simulink model "networkanalyzer"  (R2012b)
settings: Solver=ode3  SolverMode=SingleTasking  StartTime=0.0  StopTime=50000  RelTol=1e-3
libraries: xbsIndex_r4 x1097, casper_library_flow_control x33, casper_library_misc x21, xps_library x10
(part 1 of 8)
settings Model: Creator=tmadden  LastModifiedBy=tmadden

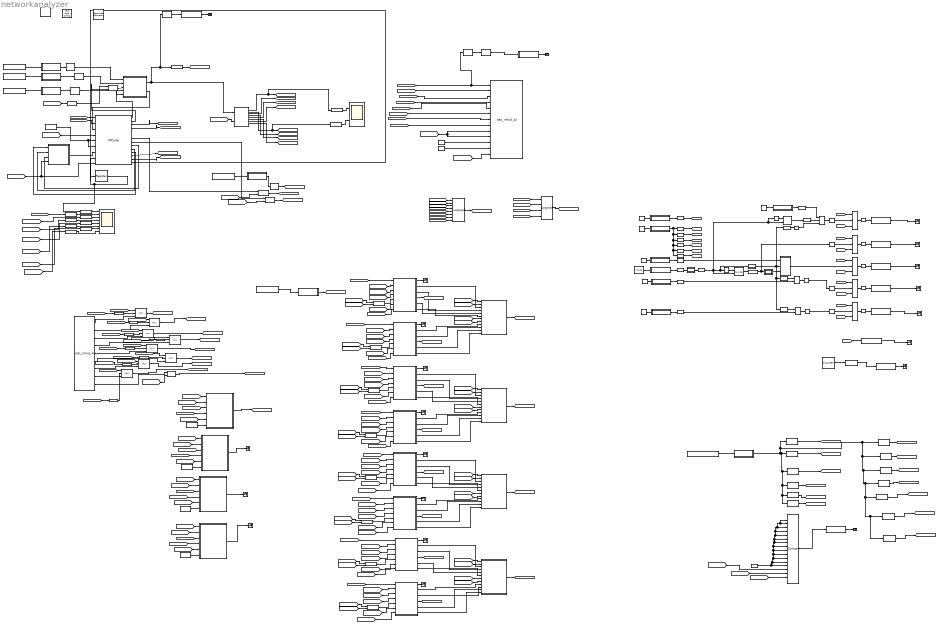
== system networkanalyzer ==
  note: The above is Ran's design for  ROACH IF baord
      | serial data stream. For programming IF board
      | clocks, gains, dividers.
  note: Signed 8 bit int
  note: Signed 8 bit, integer
  note: acc_cntrl has a clock
      | cycle latency in generating
      | new_acc signal.
      | Compensate by delaying
      | ata here.
  note: SWAT_LE
  note: LO_SLE
  note: SER_DI
  note: SER_CLK
  note: SW_STB
  note: Added by Tim Madden
  note: not in RANS design- below. Tim added the clk sle register so we can program the clocks
  note: bit 7
  note: CLK_SLE
  " System Generator" : xbsIndex_r4/ System Generator  Tag=genX  xilinxfamily=virtex5  part=xc5vsx95t  speed=-1  package=ff1136  synthesis_tool=XST  clock_wrapper=Clock Enables  directory=./networkanalyzer/sysgen  proj_type=Project Navigator  Synth_file=XST Defaults  Impl_file=ISE Defaults  testbench=off  simulink_period=1  sysclk_period=7.8125  dcm_input_clock_period=100  incr_netlist=off  trim_vbits=Everywhere in SubSystem  dbl_ovrd=According to Block Masks  core_generation=According to Block Masks  run_coregen=off  deprecated_control=off  eval_field=0  block_type=sysgen
  Concat : xbsIndex_r4/Concat  num_inputs=16  dbl_ovrd=off  block_type=concat
  Constant{,17..19} (4 alike) : xbsIndex_r4/Constant  const=0  gui_display_data_type=Boolean  arith_type=Boolean  n_bits=16  bin_pt=14  preci_type=Single  exp_width=8  frac_width=24  explicit_period=on  period=1  equ=P=C  opselect=C  inp2=PCIN>>17  opr=+  inp1=P  carry=CIN  dbl_ovrd=off  block_type=constant
  Constant1 : Constant  Value=(2^1) + (2^3) + (2^4) + (2^9)+(2^12)
  Constant10 : xbsIndex_r4/Constant  const=0  gui_display_data_type=Boolean  arith_type=Boolean  n_bits=4  bin_pt=0  preci_type=Single  exp_width=8  frac_width=24  explicit_period=on  period=1  equ=P=C  opselect=C  inp2=PCIN>>17  opr=+  inp1=P  carry=CIN  dbl_ovrd=off  block_type=constant
      settings: block_version=11.4
  Constant{11,13..15} (4 alike) : Constant
  Constant12 : Constant  Value=2^31 + 2^29 + 2^15+2^4 + 2^0
  Constant16 : Constant  Value=0
  Constant2 : Constant  Value=83886080
  Constant20 : Constant  Value=(2^26)*(64/512)
  Constant3 : Constant  Value=838860800
  Constant4 : Constant  Value=368640
  Constant5 : xbsIndex_r4/Constant  const=0  gui_display_data_type=Boolean  arith_type=Boolean  n_bits=16  bin_pt=14  preci_type=Single  exp_width=8  frac_width=24  explicit_period=off  period=1  equ=P=C  opselect=C  inp2=PCIN>>17  opr=+  inp1=P  carry=CIN  dbl_ovrd=off  block_type=constant
  Constant6 : xbsIndex_r4/Constant  const=0  gui_display_data_type=Fixed-point  arith_type=Boolean  n_bits=4  bin_pt=0  preci_type=Single  exp_width=8  frac_width=24  explicit_period=on  period=1  equ=P=C  opselect=C  inp2=PCIN>>17  opr=+  inp1=P  carry=CIN  dbl_ovrd=off  block_type=constant
      settings: block_version=11.4
  Constant8 : xbsIndex_r4/Constant  const=0  gui_display_data_type=Fixed-point  arith_type=Unsigned  n_bits=4  bin_pt=0  preci_type=Single  exp_width=8  frac_width=24  explicit_period=on  period=1  equ=P=C  opselect=C  inp2=PCIN>>17  opr=+  inp1=P  carry=CIN  dbl_ovrd=off  block_type=constant
      settings: block_version=11.4
  Constant9 : Constant  Value=512
  Convert : xbsIndex_r4/Convert  gui_display_data_type=Fixed-point  arith_type="Signed  (2's comp)"  n_bits=32  bin_pt=15  float_type=Single  exp_bits=8  fraction_bits=24  quantization=Truncate  overflow=Wrap  en=off  latency=0  dbl_ovrd=off  pipeline=off  block_type=convert
  Convert5 : xbsIndex_r4/Convert  gui_display_data_type=Fixed-point  arith_type=Unsigned  n_bits=33  bin_pt=0  float_type=Single  exp_bits=8  fraction_bits=24  quantization=Truncate  overflow=Wrap  en=off  latency=0  dbl_ovrd=off  pipeline=off  block_type=convert
      settings: block_version=11.4
  CosSinGen : Subsystem
  Counter : xbsIndex_r4/Counter  cnt_type=Free Running  cnt_to=Inf  operation=Up  start_count=0  cnt_by_val=1  arith_type=Unsigned  n_bits=24  bin_pt=0  load_pin=off  rst=off  en=off  explicit_period=on  period=1  dbl_ovrd=off  use_behavioral_HDL=off  implementation=Fabric  block_type=counter
  Counter2 : xbsIndex_r4/Counter  cnt_type=Free Running  cnt_to=2048  operation=Up  start_count=0  cnt_by_val=1  arith_type=Unsigned  n_bits=8  bin_pt=0  load_pin=off  rst=on  en=on  explicit_period=on  period=1  dbl_ovrd=off  use_behavioral_HDL=off  implementation=Fabric  use_rpm=off  block_type=counter
  Counter4 : xbsIndex_r4/Counter  cnt_type=Free Running  cnt_to=Inf  operation=Up  start_count=0  cnt_by_val=1  arith_type=Unsigned  n_bits=8  bin_pt=0  load_pin=off  rst=on  en=on  explicit_period=on  period=1  dbl_ovrd=off  use_behavioral_HDL=off  implementation=Fabric  block_type=counter
      settings: block_version=11.4
  DFTMem1 : Subsystem
  DFTMem2 : Subsystem
  DFTMem3 : Subsystem
  DFTMem4 : Subsystem
  DFTW : Subsystem
  DFTW1 : Subsystem
  DFTW2 : Subsystem
  DFTW3 : Subsystem
  DFTW4 : Subsystem
  DFTW5 : Subsystem
  DFTW6 : Subsystem
  DFTW7 : Subsystem
  Delay{1..2,9..12,29..32,34} (11 alike) : xbsIndex_r4/Delay  rst=off  infoeditControl=Selection of Reset will increase slice count due to use of real FFs and instead of SRLs  en=off  latency=1  dbl_ovrd=off  reg_retiming=off  block_type=delay
  Delay{23..24,27..28} (4 alike) : xbsIndex_r4/Delay  rst=off  infoeditControl=Selection of Reset will increase slice count due to use of real FFs and instead of SRLs  en=off  latency=64  dbl_ovrd=off  reg_retiming=off  block_type=delay
      settings: block_version=11.4
  FreqSweeper : Subsystem
  Gateway Out{1..5,7..8,12..15} (11 alike) : xbsIndex_r4/Gateway Out  inherit_from_input=off  hdl_port=off  timing_constraint=None  locs_specified=off  LOCs={}  UseAsDAC=off  DACChannel='1'  block_type=gatewayout
  Inverter{1..5} (5 alike) : xbsIndex_r4/Inverter  en=off  latency=0  dbl_ovrd=off  block_type=inv
      settings: block_version=11.4
  LO_SLE : Subsystem  Tag=xps:sw_reg  AncestorBlock=xps_library/software register  mask{numios=1, io_dir=From Processor, io_delay=0, sample_period=1, name1=reg, bitwidth1=32, arith_type1=Unsigned, bin_pt1=0}
      mask prompts: numios "Num I/Os"; io_dir "I/O direction"; io_delay "I/O delay"; sample_period "Sample period"; name1 "Name"; bitwidth1 "Bitwidth"; arith_type1 "Type"; bin_pt1 "Binary pt"
      mask init:
      | swreg_init(gcb);
      mask Callback numios: t = timer('StartDelay', 0.1); t.TimerFcn = {@swreg_cb, gcb}; start(t);
      mask TypeOptions io_dir: To Processor | From Processor
      mask Callback io_dir:
      | a = get_param(gcb, 'MaskEnables');
      | if strcmp(get_param(gcb, 'io_dir'), 'To Processor'),
      | a(4) = {'off'};
      | else
      | a(4) = {'on'};
      | end
      | set_param(gcb, 'MaskEnables', a);
      mask TypeOptions arith_type1: Unsigned | Signed  (2's comp) | Boolean
      mask Callback arith_type1:
      | a = get_param(gcb, 'MaskEnables');
      | if strcmp(get_param(gcb, 'arith_type1'), 'Boolean'),
      | set_param(gcb, 'bitwidth1', '1');
      | set_param(gcb, 'bin_pt1', '0');
      | a(6) = {'off'};
      | a(8) = {'off'};
      | else
      | a(6) = {'on'};
      | a(8) = {'on'};
      | end
      | set_param(gcb, 'MaskEnables', a);
  Logical{,1..2,17} (4 alike) : xbsIndex_r4/Logical  logical_function=OR  inputs=2  en=off  latency=0  precision=Full  arith_type=Unsigned  n_bits=16  bin_pt=0  align_bp=on  dbl_ovrd=off  block_type=logical
  Logical{3..8,10..13} (10 alike) : xbsIndex_r4/Logical  logical_function=AND  inputs=2  en=off  latency=0  precision=Full  arith_type=Unsigned  n_bits=16  bin_pt=0  align_bp=on  dbl_ovrd=off  block_type=logical
      Logical7 settings: block_version=11.4
      Logical8 settings: block_version=11.4
  Logical14 : xbsIndex_r4/Logical  logical_function=AND  inputs=8  en=off  latency=1  precision=Full  arith_type=Unsigned  n_bits=16  bin_pt=0  align_bp=on  dbl_ovrd=off  block_type=logical
  Logical15 : xbsIndex_r4/Logical  logical_function=AND  inputs=4  en=off  latency=1  precision=Full  arith_type=Unsigned  n_bits=16  bin_pt=0  align_bp=on  dbl_ovrd=off  block_type=logical
  Logical9 : xbsIndex_r4/Logical  logical_function=AND  inputs=3  en=off  latency=0  precision=Full  arith_type=Unsigned  n_bits=16  bin_pt=0  align_bp=on  dbl_ovrd=off  block_type=logical
      settings: block_version=11.4
  MainFSMScope1 : Scope  NumInputPorts=8
      settings: YMin=0~-5~-5~-5~-5~-5~-5~-5  YMax=300000~5~5~5~5~5~5~5  SaveName=ScopeData7  MaxDataPoints=10000
  MainFSMScope2 : Scope  NumInputPorts=2
      settings: YMin=0~-5  YMax=300000~5  SaveName=ScopeData2  MaxDataPoints=10000
  Mux{,1..12} (13 alike) : xbsIndex_r4/Mux  inputs=2  en=off  latency=1  precision=Full  arith_type=Unsigned  n_bits=16  bin_pt=14  quantization=Truncate  overflow=Wrap  dbl_ovrd=off  block_type=mux
      Mux2 settings: block_version=11.4
      Mux3 settings: block_version=11.4
      Mux4 settings: block_version=11.4
      Mux5 settings: block_version=11.4
      Mux6 settings: block_version=11.4
  Pulse Generator2 : DiscretePulseGenerator  Period=11000  PulseWidth=10000  PhaseDelay=100
  Resource Estimator : xbsIndex_r4/Resource Estimator  Tag=resEstTag  Slices=0  FFs=0  BRAMs=0  LUTs=0  IOBs=0  EBMs=0  TBUFs=0  xl_use_estimator_area=off  est_options=Estimate  xl_estimator_area=[392 0 0 632 0 0 0]  block_type=resource_estimator
      settings: AttributesFormatString=Resource\nEstimator
  SER_DI : Subsystem  Tag=xps:sw_reg  AncestorBlock=xps_library/software register  mask{numios=1, io_dir=From Processor, io_delay=0, sample_period=1, name1=reg, bitwidth1=32, arith_type1=Unsigned, bin_pt1=0}
      mask prompts: numios "Num I/Os"; io_dir "I/O direction"; io_delay "I/O delay"; sample_period "Sample period"; name1 "Name"; bitwidth1 "Bitwidth"; arith_type1 "Type"; bin_pt1 "Binary pt"
      mask init:
      | swreg_init(gcb);
      mask Callback numios: t = timer('StartDelay', 0.1); t.TimerFcn = {@swreg_cb, gcb}; start(t);
      mask TypeOptions io_dir: To Processor | From Processor
      mask Callback io_dir:
      | a = get_param(gcb, 'MaskEnables');
      | if strcmp(get_param(gcb, 'io_dir'), 'To Processor'),
      | a(4) = {'off'};
      | else
      | a(4) = {'on'};
      | end
      | set_param(gcb, 'MaskEnables', a);
      mask TypeOptions arith_type1: Unsigned | Signed  (2's comp) | Boolean
      mask Callback arith_type1:
      | a = get_param(gcb, 'MaskEnables');
      | if strcmp(get_param(gcb, 'arith_type1'), 'Boolean'),
      | set_param(gcb, 'bitwidth1', '1');
      | set_param(gcb, 'bin_pt1', '0');
      | a(6) = {'off'};
      | a(8) = {'off'};
      | else
      | a(6) = {'on'};
      | a(8) = {'on'};
      | end
      | set_param(gcb, 'MaskEnables', a);
  SWAT_LE : Subsystem  Tag=xps:sw_reg  AncestorBlock=xps_library/software register  mask{numios=1, io_dir=From Processor, io_delay=0, sample_period=1, name1=reg, bitwidth1=32, arith_type1=Unsigned, bin_pt1=0}
      mask prompts: numios "Num I/Os"; io_dir "I/O direction"; io_delay "I/O delay"; sample_period "Sample period"; name1 "Name"; bitwidth1 "Bitwidth"; arith_type1 "Type"; bin_pt1 "Binary pt"
      mask init:
      | swreg_init(gcb);
      mask Callback numios: t = timer('StartDelay', 0.1); t.TimerFcn = {@swreg_cb, gcb}; start(t);
      mask TypeOptions io_dir: To Processor | From Processor
      mask Callback io_dir:
      | a = get_param(gcb, 'MaskEnables');
      | if strcmp(get_param(gcb, 'io_dir'), 'To Processor'),
      | a(4) = {'off'};
      | else
      | a(4) = {'on'};
      | end
      | set_param(gcb, 'MaskEnables', a);
      mask TypeOptions arith_type1: Unsigned | Signed  (2's comp) | Boolean
      mask Callback arith_type1:
      | a = get_param(gcb, 'MaskEnables');
      | if strcmp(get_param(gcb, 'arith_type1'), 'Boolean'),
      | set_param(gcb, 'bitwidth1', '1');
      | set_param(gcb, 'bin_pt1', '0');
      | a(6) = {'off'};
      | a(8) = {'off'};
      | else
      | a(6) = {'on'};
      | a(8) = {'on'};
      | end
      | set_param(gcb, 'MaskEnables', a);
  SixFourDivLen32p26 : Subsystem  Tag=xps:sw_reg  AncestorBlock=xps_library/software register  mask{numios=1, io_dir=From Processor, io_delay=0, sample_period=1, name1=reg, bitwidth1=32, arith_type1=Unsigned, bin_pt1=0}
      mask prompts: numios "Num I/Os"; io_dir "I/O direction"; io_delay "I/O delay"; sample_period "Sample period"; name1 "Name"; bitwidth1 "Bitwidth"; arith_type1 "Type"; bin_pt1 "Binary pt"
      mask init:
      | swreg_init(gcb);
      mask Callback numios: t = timer('StartDelay', 0.1); t.TimerFcn = {@swreg_cb, gcb}; start(t);
      mask TypeOptions io_dir: To Processor | From Processor
      mask Callback io_dir:
      | a = get_param(gcb, 'MaskEnables');
      | if strcmp(get_param(gcb, 'io_dir'), 'To Processor'),
      | a(4) = {'off'};
      | else
      | a(4) = {'on'};
      | end
      | set_param(gcb, 'MaskEnables', a);
      mask TypeOptions arith_type1: Unsigned | Signed  (2's comp) | Boolean
      mask Callback arith_type1:
      | a = get_param(gcb, 'MaskEnables');
      | if strcmp(get_param(gcb, 'arith_type1'), 'Boolean'),
      | set_param(gcb, 'bitwidth1', '1');
      | set_param(gcb, 'bin_pt1', '0');
      | a(6) = {'off'};
      | a(8) = {'off'};
      | else
      | a(6) = {'on'};
      | a(8) = {'on'};
      | end
      | set_param(gcb, 'MaskEnables', a);
  Slice1 : xbsIndex_r4/Slice  nbits=1  boolean_output=on  mode=Lower Bit Location + Width  bit1=0  base1=MSB of Input  bit0=4  base0=LSB of Input  dbl_ovrd=off  block_type=slice
  Slice10 : xbsIndex_r4/Slice  nbits=1  boolean_output=on  mode=Upper Bit Location + Width  bit1=0  base1=MSB of Input  bit0=0  base0=LSB of Input  dbl_ovrd=off  block_type=slice
  Slice11 : xbsIndex_r4/Slice  nbits=1  boolean_output=on  mode=Lower Bit Location + Width  bit1=0  base1=MSB of Input  bit0=3  base0=LSB of Input  dbl_ovrd=off  block_type=slice
  Slice{14..15,20..21,26} (5 alike) : xbsIndex_r4/Slice  nbits=1  boolean_output=on  mode=Lower Bit Location + Width  bit1=0  base1=MSB of Input  bit0=0  base0=LSB of Input  dbl_ovrd=off  block_type=slice
  Slice2 : xbsIndex_r4/Slice  nbits=1  boolean_output=off  mode=Lower Bit Location + Width  bit1=0  base1=MSB of Input  bit0=0  base0=LSB of Input  dbl_ovrd=off  block_type=slice
  Slice22 : xbsIndex_r4/Slice  nbits=1  boolean_output=on  mode=Lower Bit Location + Width  bit1=0  base1=MSB of Input  bit0=1  base0=LSB of Input  dbl_ovrd=off  block_type=slice
  Slice25 : xbsIndex_r4/Slice  nbits=1  boolean_output=off  mode=Lower Bit Location + Width  bit1=0  base1=MSB of Input  bit0=2  base0=LSB of Input  dbl_ovrd=off  block_type=slice
  Slice3 : xbsIndex_r4/Slice  nbits=7  boolean_output=on  mode=Lower Bit Location + Width  bit1=0  base1=MSB of Input  bit0=0  base0=MSB of Input  dbl_ovrd=off  block_type=slice
      settings: block_version=10.1.3
  Slice4 : xbsIndex_r4/Slice  nbits=1  boolean_output=on  mode=Lower Bit Location + Width  bit1=0  base1=MSB of Input  bit0=5  base0=LSB of Input  dbl_ovrd=off  block_type=slice
  Stack4_ : Subsystem
  Terminator{,1..20} (21 alike) : Terminator
  XSG core config : xps_library/XSG core config  Tag=xps:xsg  hw_sys=ROACH:sx95t  clk_src=adc1_clk  ROACH_clk_src=adc1_clk  ROACH2_clk_src=adc0_clk  clk_rate=128  sample_period=1  synthesis_tool=XST
  adcWaveMem : Subsystem
  adcWaveMem1 : Subsystem
  adcWaveMem2 : Subsystem
  adcWaveMem3 : Subsystem
  adc_mkid_4x : xps_library/ADCs/adc_mkid_4x  Tag=xps:adc_mkid_4x  adc_brd=1  adc_clk_rate=512
  bit0 : xbsIndex_r4/Slice  nbits=1  boolean_output=on  mode=Lower Bit Location + Width  bit1=0  base1=MSB of Input  bit0=0  base0=LSB of Input  dbl_ovrd=off  block_type=slice
  bit1 : xbsIndex_r4/Slice  nbits=1  boolean_output=on  mode=Lower Bit Location + Width  bit1=0  base1=MSB of Input  bit0=1  base0=LSB of Input  dbl_ovrd=off  block_type=slice
  bit12 : xbsIndex_r4/Slice  nbits=1  boolean_output=on  mode=Lower Bit Location + Width  bit1=0  base1=MSB of Input  bit0=12  base0=LSB of Input  dbl_ovrd=off  block_type=slice
  bit13 : xbsIndex_r4/Slice  nbits=1  boolean_output=on  mode=Lower Bit Location + Width  bit1=0  base1=MSB of Input  bit0=13  base0=LSB of Input  dbl_ovrd=off  block_type=slice
  bit15 : xbsIndex_r4/Slice  nbits=1  boolean_output=on  mode=Lower Bit Location + Width  bit1=0  base1=MSB of Input  bit0=15  base0=LSB of Input  dbl_ovrd=off  block_type=slice
  bit2 : xbsIndex_r4/Slice  nbits=1  boolean_output=on  mode=Lower Bit Location + Width  bit1=0  base1=MSB of Input  bit0=2  base0=LSB of Input  dbl_ovrd=off  block_type=slice
  bit3 : xbsIndex_r4/Slice  nbits=1  boolean_output=on  mode=Lower Bit Location + Width  bit1=0  base1=MSB of Input  bit0=3  base0=LSB of Input  dbl_ovrd=off  block_type=slice
  bit4 : xbsIndex_r4/Slice  nbits=1  boolean_output=on  mode=Lower Bit Location + Width  bit1=0  base1=MSB of Input  bit0=4  base0=LSB of Input  dbl_ovrd=off  block_type=slice
  bit5 : xbsIndex_r4/Slice  nbits=1  boolean_output=on  mode=Lower Bit Location + Width  bit1=0  base1=MSB of Input  bit0=5  base0=LSB of Input  dbl_ovrd=off  block_type=slice
  bit6 : xbsIndex_r4/Slice  nbits=1  boolean_output=on  mode=Lower Bit Location + Width  bit1=0  base1=MSB of Input  bit0=6  base0=LSB of Input  dbl_ovrd=off  block_type=slice
  bit7 : xbsIndex_r4/Slice  nbits=1  boolean_output=on  mode=Lower Bit Location + Width  bit1=0  base1=MSB of Input  bit0=7  base0=LSB of Input  dbl_ovrd=off  block_type=slice
  bit8 : xbsIndex_r4/Slice  nbits=1  boolean_output=on  mode=Lower Bit Location + Width  bit1=0  base1=MSB of Input  bit0=8  base0=LSB of Input  dbl_ovrd=off  block_type=slice
  bit9__ : xbsIndex_r4/Slice  nbits=1  boolean_output=off  mode=Lower Bit Location + Width  bit1=0  base1=MSB of Input  bit0=9  base0=LSB of Input  dbl_ovrd=off  block_type=slice
  cntbit10 : xbsIndex_r4/Slice  nbits=1  boolean_output=off  mode=Lower Bit Location + Width  bit1=0  base1=LSB of Input  bit0=10  base0=LSB of Input  dbl_ovrd=off  block_type=slice
  controlReg : Subsystem  Tag=xps:sw_reg  AncestorBlock=xps_library/software register  mask{numios=1, io_dir=From Processor, io_delay=0, sample_period=1, name1=reg, bitwidth1=32, arith_type1=Unsigned, bin_pt1=0}
      mask prompts: numios "Num I/Os"; io_dir "I/O direction"; io_delay "I/O delay"; sample_period "Sample period"; name1 "Name"; bitwidth1 "Bitwidth"; arith_type1 "Type"; bin_pt1 "Binary pt"
      mask init:
      | swreg_init(gcb);
      mask Callback numios: t = timer('StartDelay', 0.1); t.TimerFcn = {@swreg_cb, gcb}; start(t);
      mask TypeOptions io_dir: To Processor | From Processor
      mask Callback io_dir:
      | a = get_param(gcb, 'MaskEnables');
      | if strcmp(get_param(gcb, 'io_dir'), 'To Processor'),
      | a(4) = {'off'};
      | else
      | a(4) = {'on'};
      | end
      | set_param(gcb, 'MaskEnables', a);
      mask TypeOptions arith_type1: Unsigned | Signed  (2's comp) | Boolean
      mask Callback arith_type1:
      | a = get_param(gcb, 'MaskEnables');
      | if strcmp(get_param(gcb, 'arith_type1'), 'Boolean'),
      | set_param(gcb, 'bitwidth1', '1');
      | set_param(gcb, 'bin_pt1', '0');
      | a(6) = {'off'};
      | a(8) = {'off'};
      | else
      | a(6) = {'on'};
      | a(8) = {'on'};
      | end
      | set_param(gcb, 'MaskEnables', a);
  currentFreq : Subsystem  Tag=xps:sw_reg  AncestorBlock=xps_library/software register  mask{numios=1, io_dir=To Processor, io_delay=0, sample_period=1, name1=reg, bitwidth1=32, arith_type1=Unsigned, bin_pt1=0}
      mask prompts: numios "Num I/Os"; io_dir "I/O direction"; io_delay "I/O delay"; sample_period "Sample period"; name1 "Name"; bitwidth1 "Bitwidth"; arith_type1 "Type"; bin_pt1 "Binary pt"
      mask init:
      | swreg_init(gcb);
      mask Callback numios: t = timer('StartDelay', 0.1); t.TimerFcn = {@swreg_cb, gcb}; start(t);
      mask TypeOptions io_dir: To Processor | From Processor
      mask Callback io_dir:
      | a = get_param(gcb, 'MaskEnables');
      | if strcmp(get_param(gcb, 'io_dir'), 'To Processor'),
      | a(4) = {'off'};
      | else
      | a(4) = {'on'};
      | end
      | set_param(gcb, 'MaskEnables', a);
      mask TypeOptions arith_type1: Unsigned | Signed  (2's comp) | Boolean
      mask Callback arith_type1:
      | a = get_param(gcb, 'MaskEnables');
      | if strcmp(get_param(gcb, 'arith_type1'), 'Boolean'),
      | set_param(gcb, 'bitwidth1', '1');
      | set_param(gcb, 'bin_pt1', '0');
      | a(6) = {'off'};
      | a(8) = {'off'};
      | else
      | a(6) = {'on'};
      | a(8) = {'on'};
      | end
      | set_param(gcb, 'MaskEnables', a);
  currentState : xbsIndex_r4/Register  init=0  rst=off  en=off  dbl_ovrd=off  block_type=register
  dac_mkid_4x : xps_library/DACs/dac_mkid_4x  Tag=xps:dac_mkid_4x  dac_brd=0  dac_clk_rate=512  sample_period=1
  dftLen : Subsystem  Tag=xps:sw_reg  AncestorBlock=xps_library/software register  mask{numios=1, io_dir=From Processor, io_delay=0, sample_period=1, name1=reg, bitwidth1=32, arith_type1=Unsigned, bin_pt1=0}
      mask prompts: numios "Num I/Os"; io_dir "I/O direction"; io_delay "I/O delay"; sample_period "Sample period"; name1 "Name"; bitwidth1 "Bitwidth"; arith_type1 "Type"; bin_pt1 "Binary pt"
      mask init:
      | swreg_init(gcb);
      mask Callback numios: t = timer('StartDelay', 0.1); t.TimerFcn = {@swreg_cb, gcb}; start(t);
      mask TypeOptions io_dir: To Processor | From Processor
      mask Callback io_dir:
      | a = get_param(gcb, 'MaskEnables');
      | if strcmp(get_param(gcb, 'io_dir'), 'To Processor'),
      | a(4) = {'off'};
      | else
      | a(4) = {'on'};
      | end
      | set_param(gcb, 'MaskEnables', a);
      mask TypeOptions arith_type1: Unsigned | Signed  (2's comp) | Boolean
      mask Callback arith_type1:
      | a = get_param(gcb, 'MaskEnables');
      | if strcmp(get_param(gcb, 'arith_type1'), 'Boolean'),
      | set_param(gcb, 'bitwidth1', '1');
      | set_param(gcb, 'bin_pt1', '0');
      | a(6) = {'off'};
      | a(8) = {'off'};
      | else
      | a(6) = {'on'};
      | a(8) = {'on'};
      | end
      | set_param(gcb, 'MaskEnables', a);
  edge_detect : casper_library_misc/edge_detect  edge=Rising  polarity=Active High  x_in=[0 0.08 0.08 0.16 0.16 0.24 0.24 0.32 0.32 0.4]  y_in="[-1 -1  1  1  1  1  1  1  1  1]"  x_out=[0.6 0.68 0.68 0.76 0.76 0.84 0.84 0.92 0.92 1]  y_out="[-1 -1  1  1 -1 -1 -1 -1 -1 -1]"
  endFreq : Subsystem  Tag=xps:sw_reg  AncestorBlock=xps_library/software register  mask{numios=1, io_dir=From Processor, io_delay=0, sample_period=1, name1=reg, bitwidth1=32, arith_type1=Unsigned, bin_pt1=0}
      mask prompts: numios "Num I/Os"; io_dir "I/O direction"; io_delay "I/O delay"; sample_period "Sample period"; name1 "Name"; bitwidth1 "Bitwidth"; arith_type1 "Type"; bin_pt1 "Binary pt"
      mask init:
      | swreg_init(gcb);
      mask Callback numios: t = timer('StartDelay', 0.1); t.TimerFcn = {@swreg_cb, gcb}; start(t);
      mask TypeOptions io_dir: To Processor | From Processor
      mask Callback io_dir:
      | a = get_param(gcb, 'MaskEnables');
      | if strcmp(get_param(gcb, 'io_dir'), 'To Processor'),
      | a(4) = {'off'};
      | else
      | a(4) = {'on'};
      | end
      | set_param(gcb, 'MaskEnables', a);
      mask TypeOptions arith_type1: Unsigned | Signed  (2's comp) | Boolean
      mask Callback arith_type1:
      | a = get_param(gcb, 'MaskEnables');
      | if strcmp(get_param(gcb, 'arith_type1'), 'Boolean'),
      | set_param(gcb, 'bitwidth1', '1');
      | set_param(gcb, 'bin_pt1', '0');
      | a(6) = {'off'};
      | a(8) = {'off'};
      | else
      | a(6) = {'on'};
      | a(8) = {'on'};
      | end
      | set_param(gcb, 'MaskEnables', a);
  fix12_11_{,1..7} (8 alike) : xbsIndex_r4/Convert  gui_display_data_type=Fixed-point  arith_type="Signed  (2's comp)"  n_bits=12  bin_pt=11  float_type=Single  exp_bits=8  fraction_bits=24  quantization=Truncate  overflow=Saturate  en=off  latency=0  dbl_ovrd=off  pipeline=off  block_type=convert
  freqAddend : Subsystem  Tag=xps:sw_reg  AncestorBlock=xps_library/software register  mask{numios=1, io_dir=From Processor, io_delay=0, sample_period=1, name1=reg, bitwidth1=32, arith_type1=Unsigned, bin_pt1=0}
      mask prompts: numios "Num I/Os"; io_dir "I/O direction"; io_delay "I/O delay"; sample_period "Sample period"; name1 "Name"; bitwidth1 "Bitwidth"; arith_type1 "Type"; bin_pt1 "Binary pt"
      mask init:
      | swreg_init(gcb);
      mask Callback numios: t = timer('StartDelay', 0.1); t.TimerFcn = {@swreg_cb, gcb}; start(t);
      mask TypeOptions io_dir: To Processor | From Processor
      mask Callback io_dir:
      | a = get_param(gcb, 'MaskEnables');
      | if strcmp(get_param(gcb, 'io_dir'), 'To Processor'),
      | a(4) = {'off'};
      | else
      | a(4) = {'on'};
      | end
      | set_param(gcb, 'MaskEnables', a);
      mask TypeOptions arith_type1: Unsigned | Signed  (2's comp) | Boolean
      mask Callback arith_type1:
      | a = get_param(gcb, 'MaskEnables');
      | if strcmp(get_param(gcb, 'arith_type1'), 'Boolean'),
      | set_param(gcb, 'bitwidth1', '1');
      | set_param(gcb, 'bin_pt1', '0');
      | a(6) = {'off'};
      | a(8) = {'off'};
      | else
      | a(6) = {'on'};
      | a(8) = {'on'};
      | end
      | set_param(gcb, 'MaskEnables', a);
  gpio_a0 : xps_library/gpio  Tag=xps:gpio  io_group=ROACH:gpioa  io_dir=out  arith_type=Unsigned  bitwidth=1  bin_pt=0  bit_index=3  sample_period=1  use_single_ended=off  use_ddr=off  reg_iob=on  reg_clk_phase=0  termination=None
  gpio_a1 : xps_library/gpio  Tag=xps:gpio  io_group=ROACH:gpioa  io_dir=out  arith_type=Unsigned  bitwidth=1  bin_pt=0  bit_index=2  sample_period=1  use_single_ended=off  use_ddr=off  reg_iob=on  reg_clk_phase=0  termination=None
  gpio_a2 : xps_library/gpio  Tag=xps:gpio  io_group=ROACH:gpioa  io_dir=out  arith_type=Unsigned  bitwidth=1  bin_pt=0  bit_index=1  sample_period=1  use_single_ended=off  use_ddr=off  reg_iob=on  reg_clk_phase=0  termination=None
  gpio_a3 : xps_library/gpio  Tag=xps:gpio  io_group=ROACH:gpioa  io_dir=out  arith_type=Unsigned  bitwidth=1  bin_pt=0  bit_index=0  sample_period=1  use_single_ended=off  use_ddr=off  reg_iob=on  reg_clk_phase=0  termination=None
  gpio_a4 : xps_library/gpio  Tag=xps:gpio  io_group=ROACH:gpioa  io_dir=out  arith_type=Unsigned  bitwidth=1  bin_pt=0  bit_index=7  sample_period=1  use_single_ended=off  use_ddr=off  reg_iob=on  reg_clk_phase=0  termination=None
  gpio_a5 : xps_library/gpio  Tag=xps:gpio  io_group=ROACH:gpioa  io_dir=out  arith_type=Unsigned  bitwidth=1  bin_pt=0  bit_index=6  sample_period=1  use_single_ended=off  use_ddr=off  reg_iob=on  reg_clk_phase=0  termination=None
  gpio_a7 : xps_library/gpio  Tag=xps:gpio  io_group=ROACH:gpioa  io_dir=out  arith_type=Unsigned  bitwidth=1  bin_pt=0  bit_index=4  sample_period=1  use_single_ended=off  use_ddr=off  reg_iob=on  reg_clk_phase=0  termination=None
  if_switch : Subsystem  Tag=xps:sw_reg  AncestorBlock=xps_library/software register  mask{numios=1, io_dir=From Processor, io_delay=0, sample_period=1, name1=reg, bitwidth1=32, arith_type1=Unsigned, bin_pt1=0}
      mask prompts: numios "Num I/Os"; io_dir "I/O direction"; io_delay "I/O delay"; sample_period "Sample period"; name1 "Name"; bitwidth1 "Bitwidth"; arith_type1 "Type"; bin_pt1 "Binary pt"
      mask init:
      | swreg_init(gcb);
      mask Callback numios: t = timer('StartDelay', 0.1); t.TimerFcn = {@swreg_cb, gcb}; start(t);
      mask TypeOptions io_dir: To Processor | From Processor
      mask Callback io_dir:
      | a = get_param(gcb, 'MaskEnables');
      | if strcmp(get_param(gcb, 'io_dir'), 'To Processor'),
      | a(4) = {'off'};
      | else
      | a(4) = {'on'};
      | end
      | set_param(gcb, 'MaskEnables', a);
      mask TypeOptions arith_type1: Unsigned | Signed  (2's comp) | Boolean
      mask Callback arith_type1:
      | a = get_param(gcb, 'MaskEnables');
      | if strcmp(get_param(gcb, 'arith_type1'), 'Boolean'),
      | set_param(gcb, 'bitwidth1', '1');
      | set_param(gcb, 'bin_pt1', '0');
      | a(6) = {'off'};
      | a(8) = {'off'};
      | else
      | a(6) = {'on'};
      | a(8) = {'on'};
      | end
      | set_param(gcb, 'MaskEnables', a);
  mainFSM : xbsIndex_r4/MCode  mfname=mainFSM  explicit_period=on  period=1  inputsTable={'boundInpExpr'=>['userMemDone','dftDone','isEndFreq','trigSweepDFT','trigSweep','setConstFreq','popdata','state','rst'],'inputs'=>['userMemDone','dftDone','isEndFreq','trigSweepDFT','trigSweep','setConstFreq','popdata','state','rst']}  outputsTable={'outputs'=>['rstStartFreq','incFreq','wrUserMem1','wrUserMem','isSweeping','idleStby','clrDFT','dValidDFT','pop','push','pushdata','userMemStrt','userMemSel','nextstate'],'suppressOut'=>['off','off','off','off','off','off','off','off','off','off','off','off','off','off']}  dbl_ovrd=off  enable_stdout=on  enable_debug=off  suppress_output=on  defparams={'userMemDone',userMemDone,'dftDone',dftDone,'isEndFreq',isEndFreq,'trigSweepDFT',trigSweepDFT,'trigSweep',trigSweep,'setConstFreq',setConstFreq,'popdata',popdata,'state',state,'rst',rst}  hide_port_list={}  block_type=mcode
  parallel_to_serial_converter1 : Subsystem  mask(parallel_to_serial_converter){pin_width=33, sout_width=1}
      mask prompts: pin_width "Parallel Input Width"; sout_width "Serial Output Width"
      mask help:
      | This block takes as input a parallel bus of specified width.
      | When the load signal 'ld' is asserted, this data is broken into
      | pieces of width specified by the serial output width and
      | stored into different registers chained to form a shift register.
      | If the 'shift' input is subsequently asserted, the shift register
      | returns as output a new piece of data of width sout_width.  This data
      | is the next least significant piece of the original bus.  The converter
      | serializes SMALL ENDIAN.
      |
      | Note that the load operation automatically loads the least significant
      | bits into the register closest to the output, so the first 'shift'
      | assertion changes the data output from bits [sout_width-1:0] to
      | bits [2*sout_width-1:sout_width].
      mask init:
      | parallel_to_serial_converter_init(gcb, ...
      |     'pin_width', pin_width, ...
      |     'sout_width', sout_width);
  posedge2 : Subsystem  Tag=Rising Edge Detector  mask(posedge){}
      mask help: Outputs true if a boolean input signal is true this clock and was false last clock.
      mask Help: eval('xlWeb([getenv(''MLIB_ROOT''), ''\doc\htmlblocks\sp_posedge\sp_posedge.html''])')
  posedge5 : Subsystem  Tag=Rising Edge Detector  mask(posedge){}
      mask help: Outputs true if a boolean input signal is true this clock and was false last clock.
      mask Help: eval('xlWeb([getenv(''MLIB_ROOT''), ''\doc\htmlblocks\sp_posedge\sp_posedge.html''])')
  posedge6 : Subsystem  Tag=Rising Edge Detector  mask(posedge){}
      mask help: Outputs true if a boolean input signal is true this clock and was false last clock.
      mask Help: eval('xlWeb([getenv(''MLIB_ROOT''), ''\doc\htmlblocks\sp_posedge\sp_posedge.html''])')
  pulse_ext2 : casper_library_misc/pulse_ext  pulse_len=(34)*2^8
  pulse_ext3 : casper_library_misc/pulse_ext  pulse_len=(32)*2^8 + 2^7
  pulse_ext4 : casper_library_misc/pulse_ext  pulse_len=(18)*2^8 + 2^7
  pulse_ext5 : casper_library_misc/pulse_ext  pulse_len=(27)*2^8
  regs : Subsystem  Tag=xps:sw_reg  AncestorBlock=xps_library/software register  mask{numios=1, io_dir=From Processor, io_delay=0, sample_period=1, name1=reg, bitwidth1=32, arith_type1=Unsigned, bin_pt1=0}
      mask prompts: numios "Num I/Os"; io_dir "I/O direction"; io_delay "I/O delay"; sample_period "Sample period"; name1 "Name"; bitwidth1 "Bitwidth"; arith_type1 "Type"; bin_pt1 "Binary pt"
      mask init:
      | swreg_init(gcb);
      mask Callback numios: t = timer('StartDelay', 0.1); t.TimerFcn = {@swreg_cb, gcb}; start(t);
      mask TypeOptions io_dir: To Processor | From Processor
      mask Callback io_dir:
      | a = get_param(gcb, 'MaskEnables');
      | if strcmp(get_param(gcb, 'io_dir'), 'To Processor'),
      | a(4) = {'off'};
      | else
      | a(4) = {'on'};
      | end
      | set_param(gcb, 'MaskEnables', a);
      mask TypeOptions arith_type1: Unsigned | Signed  (2's comp) | Boolean
      mask Callback arith_type1:
      | a = get_param(gcb, 'MaskEnables');
      | if strcmp(get_param(gcb, 'arith_type1'), 'Boolean'),
      | set_param(gcb, 'bitwidth1', '1');
      | set_param(gcb, 'bin_pt1', '0');
      | a(6) = {'off'};
      | a(8) = {'off'};
      | else
      | a(6) = {'on'};
      | a(8) = {'on'};
      | end
      | set_param(gcb, 'MaskEnables', a);
  sineNumber : Subsystem  Tag=xps:sw_reg  AncestorBlock=xps_library/software register  mask{numios=1, io_dir=To Processor, io_delay=0, sample_period=1, name1=reg, bitwidth1=32, arith_type1=Unsigned, bin_pt1=0}
      mask prompts: numios "Num I/Os"; io_dir "I/O direction"; io_delay "I/O delay"; sample_period "Sample period"; name1 "Name"; bitwidth1 "Bitwidth"; arith_type1 "Type"; bin_pt1 "Binary pt"
      mask init:
      | swreg_init(gcb);
      mask Callback numios: t = timer('StartDelay', 0.1); t.TimerFcn = {@swreg_cb, gcb}; start(t);
      mask TypeOptions io_dir: To Processor | From Processor
      mask Callback io_dir:
      | a = get_param(gcb, 'MaskEnables');
      | if strcmp(get_param(gcb, 'io_dir'), 'To Processor'),
      | a(4) = {'off'};
      | else
      | a(4) = {'on'};
      | end
      | set_param(gcb, 'MaskEnables', a);
      mask TypeOptions arith_type1: Unsigned | Signed  (2's comp) | Boolean
      mask Callback arith_type1:
      | a = get_param(gcb, 'MaskEnables');
      | if strcmp(get_param(gcb, 'arith_type1'), 'Boolean'),
      | set_param(gcb, 'bitwidth1', '1');
      | set_param(gcb, 'bin_pt1', '0');
      | a(6) = {'off'};
      | a(8) = {'off'};
      | else
      | a(6) = {'on'};
      | a(8) = {'on'};
      | end
      | set_param(gcb, 'MaskEnables', a);
  start : Subsystem  Tag=xps:sw_reg  AncestorBlock=xps_library/software register  mask{numios=1, io_dir=From Processor, io_delay=0, sample_period=1, name1=reg, bitwidth1=32, arith_type1=Unsigned, bin_pt1=0}
      mask prompts: numios "Num I/Os"; io_dir "I/O direction"; io_delay "I/O delay"; sample_period "Sample period"; name1 "Name"; bitwidth1 "Bitwidth"; arith_type1 "Type"; bin_pt1 "Binary pt"
      mask init:
      | swreg_init(gcb);
      mask Callback numios: t = timer('StartDelay', 0.1); t.TimerFcn = {@swreg_cb, gcb}; start(t);
      mask TypeOptions io_dir: To Processor | From Processor
      mask Callback io_dir:
      | a = get_param(gcb, 'MaskEnables');
      | if strcmp(get_param(gcb, 'io_dir'), 'To Processor'),
      | a(4) = {'off'};
      | else
      | a(4) = {'on'};
      | end
      | set_param(gcb, 'MaskEnables', a);
      mask TypeOptions arith_type1: Unsigned | Signed  (2's comp) | Boolean
      mask Callback arith_type1:
      | a = get_param(gcb, 'MaskEnables');
      | if strcmp(get_param(gcb, 'arith_type1'), 'Boolean'),
      | set_param(gcb, 'bitwidth1', '1');
      | set_param(gcb, 'bin_pt1', '0');
      | a(6) = {'off'};
      | a(8) = {'off'};
      | else
      | a(6) = {'on'};
      | a(8) = {'on'};
      | end
      | set_param(gcb, 'MaskEnables', a);
  startFreq : Subsystem  Tag=xps:sw_reg  AncestorBlock=xps_library/software register  mask{numios=1, io_dir=From Processor, io_delay=0, sample_period=1, name1=reg, bitwidth1=32, arith_type1=Unsigned, bin_pt1=0}
      mask prompts: numios "Num I/Os"; io_dir "I/O direction"; io_delay "I/O delay"; sample_period "Sample period"; name1 "Name"; bitwidth1 "Bitwidth"; arith_type1 "Type"; bin_pt1 "Binary pt"
      mask init:
      | swreg_init(gcb);
      mask Callback numios: t = timer('StartDelay', 0.1); t.TimerFcn = {@swreg_cb, gcb}; start(t);
      mask TypeOptions io_dir: To Processor | From Processor
      mask Callback io_dir:
      | a = get_param(gcb, 'MaskEnables');
      | if strcmp(get_param(gcb, 'io_dir'), 'To Processor'),
      | a(4) = {'off'};
      | else
      | a(4) = {'on'};
      | end
      | set_param(gcb, 'MaskEnables', a);
      mask TypeOptions arith_type1: Unsigned | Signed  (2's comp) | Boolean
      mask Callback arith_type1:
      | a = get_param(gcb, 'MaskEnables');
      | if strcmp(get_param(gcb, 'arith_type1'), 'Boolean'),
      | set_param(gcb, 'bitwidth1', '1');
      | set_param(gcb, 'bin_pt1', '0');
      | a(6) = {'off'};
      | a(8) = {'off'};
      | else
      | a(6) = {'on'};
      | a(8) = {'on'};
      | end
      | set_param(gcb, 'MaskEnables', a);
  statusFlags : Subsystem  Tag=xps:sw_reg  AncestorBlock=xps_library/software register  mask{numios=1, io_dir=To Processor, io_delay=0, sample_period=1, name1=reg, bitwidth1=32, arith_type1=Unsigned, bin_pt1=0}
      mask prompts: numios "Num I/Os"; io_dir "I/O direction"; io_delay "I/O delay"; sample_period "Sample period"; name1 "Name"; bitwidth1 "Bitwidth"; arith_type1 "Type"; bin_pt1 "Binary pt"
      mask init:
      | swreg_init(gcb);
      mask Callback numios: t = timer('StartDelay', 0.1); t.TimerFcn = {@swreg_cb, gcb}; start(t);
      mask TypeOptions io_dir: To Processor | From Processor
      mask Callback io_dir:
      | a = get_param(gcb, 'MaskEnables');
      | if strcmp(get_param(gcb, 'io_dir'), 'To Processor'),
      | a(4) = {'off'};
      | else
      | a(4) = {'on'};
      | end
      | set_param(gcb, 'MaskEnables', a);
      mask TypeOptions arith_type1: Unsigned | Signed  (2's comp) | Boolean
      mask Callback arith_type1:
      | a = get_param(gcb, 'MaskEnables');
      | if strcmp(get_param(gcb, 'arith_type1'), 'Boolean'),
      | set_param(gcb, 'bitwidth1', '1');
      | set_param(gcb, 'bin_pt1', '0');
      | a(6) = {'off'};
      | a(8) = {'off'};
      | else
      | a(6) = {'on'};
      | a(8) = {'on'};
      | end
      | set_param(gcb, 'MaskEnables', a);
  stb_en : Subsystem  Tag=xps:sw_reg  AncestorBlock=xps_library/software register  mask{numios=1, io_dir=From Processor, io_delay=0, sample_period=1, name1=reg, bitwidth1=32, arith_type1=Unsigned, bin_pt1=0}
      mask prompts: numios "Num I/Os"; io_dir "I/O direction"; io_delay "I/O delay"; sample_period "Sample period"; name1 "Name"; bitwidth1 "Bitwidth"; arith_type1 "Type"; bin_pt1 "Binary pt"
      mask init:
      | swreg_init(gcb);
      mask Callback numios: t = timer('StartDelay', 0.1); t.TimerFcn = {@swreg_cb, gcb}; start(t);
      mask TypeOptions io_dir: To Processor | From Processor
      mask Callback io_dir:
      | a = get_param(gcb, 'MaskEnables');
      | if strcmp(get_param(gcb, 'io_dir'), 'To Processor'),
      | a(4) = {'off'};
      | else
      | a(4) = {'on'};
      | end
      | set_param(gcb, 'MaskEnables', a);
      mask TypeOptions arith_type1: Unsigned | Signed  (2's comp) | Boolean
      mask Callback arith_type1:
      | a = get_param(gcb, 'MaskEnables');
      | if strcmp(get_param(gcb, 'arith_type1'), 'Boolean'),
      | set_param(gcb, 'bitwidth1', '1');
      | set_param(gcb, 'bin_pt1', '0');
      | a(6) = {'off'};
      | a(8) = {'off'};
      | else
      | a(6) = {'on'};
      | a(8) = {'on'};
      | end
      | set_param(gcb, 'MaskEnables', a);
  wires:
  bit0/1 -> [mainRst]
  Gateway Out4/1 -> [curfreq]
  bit2/1 -> [manualSweep]
  bit3/1 -> [sigmaDeltaEn]
  bit4/1 -> [startDac]
  bit5/1 -> [manDFT]
  Constant1/1 -> controlReg/1(sim_reg)
  Constant2/1 -> startFreq/1(sim_reg)
  Constant3/1 -> endFreq/1(sim_reg)
  Constant4/1 -> freqAddend/1(sim_reg)
  Delay10/1 -> FreqSweeper/1(startFreq)
  Delay11/1 -> FreqSweeper/2(endFreq)
  Delay12/1 -> FreqSweeper/4(fregAddend)
  Constant9/1 -> dftLen/1(sim_reg)
  mainFSM/7 -> Logical2/1
  mainFSM/8 -> Logical1/1
  mainFSM/2 -> Logical/2
  mainFSM/1 -> FreqSweeper/5(rstFreq)
  [sigmaDeltaEn] -> CosSinGen/2(SDMen)
  Stack4_/1(DataOut) -> mainFSM/7
  mainFSM/11 -> Stack4_/1(dataIn)
  mainFSM/10 -> Stack4_/2(Push)
  mainFSM/9 -> Stack4_/3(Pop)
  FreqSweeper/2(isLastFreq) -> mainFSM/3
  bit1/1 -> [trigDftSweep]
  [mainRst] -> mainFSM/9, Stack4_/4(Rst)
  [trigDftSweep] -> mainFSM/4
  Constant5/1 -> mainFSM/6, mainFSM/5
  FreqSweeper/1(outFreq) -> CosSinGen/1(Freq), Delay2/1, Gateway Out4/1
  mainFSM/14 -> currentState/1
  mainFSM/3 -> [dftmemWE1]
  Constant6/1 -> dac_mkid_4x/11
  Constant8/1 -> dac_mkid_4x/12
  currentState/1 -> Gateway Out1/1, mainFSM/8
  startFreq/1(in_reg) -> Delay10/1
  endFreq/1(in_reg) -> Delay11/1
  freqAddend/1(in_reg) -> Delay12/1
  dftLen/1(in_reg) -> Delay9/1
  currentFreq/1(sim_out) -> Terminator2/1
  Delay2/1 -> currentFreq/1(out_reg)
  Convert5/1 -> parallel_to_serial_converter1/1(pin)
  Constant11/1 -> stb_en/1(sim_reg)
  Pulse Generator2/1 -> start/1(sim_reg)
  stb_en/1(in_reg) -> Slice15/1
  Slice14/1 -> Logical8/2
  SWAT_LE/1(in_reg) -> Slice14/1
  Inverter3/1 -> Delay28/1
  Logical8/1 -> Inverter3/1
  pulse_ext4/1 -> Logical8/1
  Slice21/1 -> Logical7/2
  Inverter1/1 -> Delay27/1
  Logical7/1 -> Inverter1/1
  LO_SLE/1(in_reg) -> Slice21/1
  pulse_ext3/1 -> Logical7/1
  Constant12/1 -> SER_DI/1(sim_reg)
  posedge6/1(Out) -> parallel_to_serial_converter1/3(shift)
  Slice26/1 -> posedge2/1(In)
  Inverter5/1 -> Counter2/1
  Counter2/1 -> Slice3/1
  Slice3/1 -> posedge6/1(In), Delay24/1
  Logical9/1 -> Delay23/1
  Counter4/1 -> Slice10/1
  Slice10/1 -> Logical9/2
  pulse_ext5/1 -> Inverter2/1
  Inverter2/1 -> Logical9/3
  Constant14/1 -> LO_SLE/1(sim_reg)
  Constant15/1 -> SWAT_LE/1(sim_reg)
  Inverter4/1 -> Counter4/1
  start/1(in_reg) -> Slice26/1
  posedge2/1(Out) -> pulse_ext2/1
  pulse_ext2/1 -> Counter2/2, Counter4/2, Inverter4/1, Inverter5/1, posedge5/1(In)
  posedge5/1(Out) -> parallel_to_serial_converter1/2(ld), pulse_ext5/1, pulse_ext3/1, pulse_ext4/1
  Delay23/1 -> Mux2/2
  Mux2/1 -> Delay34/1
  parallel_to_serial_converter1/1(sout) -> Mux3/2
  Mux3/1 -> Delay30/1
  Delay28/1 -> Mux4/2
  Mux4/1 -> Delay32/1
  Delay27/1 -> Mux5/2
  Delay24/1 -> Mux6/2
  Mux6/1 -> Delay29/1
  Mux5/1 -> Delay31/1
  Constant16/1 -> if_switch/1(sim_reg)
  if_switch/1(in_reg) -> Slice2/1
  Slice2/1 -> [if_switch]
  [if_switch] -> Mux2/1
  [if_switch] -> Mux6/1
  [if_switch] -> Mux3/1
  [if_switch] -> Mux5/1
  [if_switch] -> Mux4/1
  Constant13/1 -> regs/1(sim_reg)
  regs/1(in_reg) -> Slice20/1, Slice22/1, Slice25/1, Slice11/1, Slice4/1, Slice1/1
  Slice22/1 -> [ser_clk]
  Slice20/1 -> [sw_stb]
  Slice25/1 -> [ser_di]
  Slice11/1 -> [lo_sle]
  Slice1/1 -> [swat_le]
  [sw_stb] -> Mux2/3
  [ser_clk] -> Mux6/3
  [ser_di] -> Mux3/3
  [lo_sle] -> Mux5/3
  [swat_le] -> Mux4/3
  Delay34/1 -> gpio_a0/1
  Delay29/1 -> gpio_a1/1
  Delay30/1 -> gpio_a2/1
  Delay31/1 -> gpio_a3/1
  Delay32/1 -> gpio_a5/1
  SER_DI/1(in_reg) -> Convert5/1
  Slice15/1 -> Logical9/1
  gpio_a0/1 -> Terminator/1
  gpio_a1/1 -> Terminator3/1
  gpio_a2/1 -> Terminator4/1
  gpio_a3/1 -> Terminator5/1
  gpio_a5/1 -> Terminator6/1
  Slice4/1 -> [clk_sle]
  gpio_a4/1 -> Terminator7/1
  [clk_sle] -> gpio_a4/1
  CosSinGen/7(Cos3) -> [cos3]
  CosSinGen/8(nSin3) -> [sin3]
  CosSinGen/3(Cos1) -> [cos1]
  CosSinGen/5(Cos2) -> [cos2]
  CosSinGen/4(nSin1) -> [sin1]
  CosSinGen/6(nSin2) -> [sin2]
  Logical/1 -> FreqSweeper/3(incFreq)
  edge_detect/1 -> Logical/1
  [manualSweep] -> edge_detect/1
  [startDac] -> dac_mkid_4x/10, dac_mkid_4x/9
  statusFlags/1(sim_out) -> Terminator8/1
  Concat/1 -> statusFlags/1(out_reg)
  [dftmemDoneAll] -> Concat/16
  Constant10/1 -> Concat/1, Concat/2, Concat/3, Concat/4, Concat/5, Concat/6, Concat/7, Concat/8, Concat/9, Concat/10, Concat/11, Concat/12, Concat/13
  [manDFT] -> Logical1/2
  [clearDFT] -> Logical2/2
  bit6/1 -> [clearDFT]
  CosSinGen/1(Cos0) -> Gateway Out2/1, [cos0]
  CosSinGen/2(nSin0) -> Gateway Out3/1, [sin0]
  Logical1/1 -> [dftvalid]
  Delay9/1 -> [dftlen]
  Logical2/1 -> [dftclr]
  [dftlen] -> DFTW/3(DFTLen)
  [dftclr] -> DFTW/4(Clear)
  [cos3] -> DFTW/2(CosIn)
  [sin3] -> DFTW/6(SinIn)
  [dftlen] -> DFTW1/3(DFTLen)
  [dftclr] -> DFTW1/4(Clear)
  [cos3] -> DFTW1/2(CosIn)
  [sin3] -> DFTW1/6(SinIn)
  [dftlen] -> DFTW2/3(DFTLen)
  [dftclr] -> DFTW2/4(Clear)
  [cos0] -> DFTW2/2(CosIn)
  [sin0] -> DFTW2/6(SinIn)
  [dftlen] -> DFTW3/3(DFTLen)
  [dftclr] -> DFTW3/4(Clear)
  [cos0] -> DFTW3/2(CosIn)
  [sin0] -> DFTW3/6(SinIn)
  [dftlen] -> DFTW4/3(DFTLen)
  [dftclr] -> DFTW4/4(Clear)
  [cos1] -> DFTW4/2(CosIn)
  [sin1] -> DFTW4/6(SinIn)
  [dftlen] -> DFTW5/3(DFTLen)
  [dftclr] -> DFTW5/4(Clear)
  [cos1] -> DFTW5/2(CosIn)
  [sin1] -> DFTW5/6(SinIn)
  [dftlen] -> DFTW6/3(DFTLen)
  [dftclr] -> DFTW6/4(Clear)
  [cos2] -> DFTW6/2(CosIn)
  [sin2] -> DFTW6/6(SinIn)
  [dftlen] -> DFTW7/3(DFTLen)
  [dftclr] -> DFTW7/4(Clear)
  [cos2] -> DFTW7/2(CosIn)
  [sin2] -> DFTW7/6(SinIn)
  Mux9/1 -> [adc_q0]
  Mux1/1 -> [adc_i1]
  Mux10/1 -> [adc_q1]
  Mux7/1 -> [adc_i2]
  Mux8/1 -> [adc_i3]
  DFTW/2(ImagOutRawLo) -> DFTMem1/3(Src0)
  DFTW/3(RealOutRawLo) -> DFTMem1/4(Src1)
  DFTW/5(ImagOutRawHi) -> DFTMem1/5(Src2)
  DFTW/6(RealOutRawHi) -> DFTMem1/6(Src3)
  DFTW1/2(ImagOutRawLo) -> DFTMem1/9(Src4)
  DFTW1/3(RealOutRawLo) -> DFTMem1/10(Src5)
  DFTW1/5(ImagOutRawHi) -> DFTMem1/11(Src6)
  DFTW1/6(RealOutRawHi) -> DFTMem1/12(Src7)
  Logical17/1 -> [adcvalid]
  Logical3/1 -> DFTW3/5(ValidIn)
  [dftvalid] -> Logical3/1
  [adcvalid] -> Logical3/2
  Logical4/1 -> DFTW4/5(ValidIn)
  [dftvalid] -> Logical4/1
  [adcvalid] -> Logical4/2
  Logical5/1 -> DFTW/5(ValidIn)
  [dftvalid] -> Logical5/1
  [adcvalid] -> Logical5/2
  Logical6/1 -> DFTW1/5(ValidIn)
  [dftvalid] -> Logical6/1
  [adcvalid] -> Logical6/2
  Logical10/1 -> DFTW2/5(ValidIn)
  [dftvalid] -> Logical10/1
  [adcvalid] -> Logical10/2
  Logical11/1 -> DFTW5/5(ValidIn)
  [dftvalid] -> Logical11/1
  [adcvalid] -> Logical11/2
  Logical12/1 -> DFTW6/5(ValidIn)
  [dftvalid] -> Logical12/1
  [adcvalid] -> Logical12/2
  Logical13/1 -> DFTW7/5(ValidIn)
  [dftvalid] -> Logical13/1
  [adcvalid] -> Logical13/2
  DFTW/1(ValidPulse) -> Terminator9/1
  DFTW/4(ValiidFlag) -> [dftvalid0]
  DFTW1/1(ValidPulse) -> Terminator10/1
  DFTW1/4(ValiidFlag) -> [dftvalid1]
  [dftmemWE] -> DFTMem1/7(WE)
  [dftmemWE1] -> DFTMem1/8(WE1)
  [dftmemSel] -> DFTMem1/2(Sel)
  [dftmemStart] -> DFTMem1/1(Start)
  DFTMem1/1(Out1) -> [dftmemDone0]
  DFTW2/2(ImagOutRawLo) -> DFTMem2/3(Src0)
  DFTW2/3(RealOutRawLo) -> DFTMem2/4(Src1)
  DFTW2/5(ImagOutRawHi) -> DFTMem2/5(Src2)
  DFTW2/6(RealOutRawHi) -> DFTMem2/6(Src3)
  DFTW3/2(ImagOutRawLo) -> DFTMem2/9(Src4)
  DFTW3/3(RealOutRawLo) -> DFTMem2/10(Src5)
  DFTW3/5(ImagOutRawHi) -> DFTMem2/11(Src6)
  DFTW3/6(RealOutRawHi) -> DFTMem2/12(Src7)
  DFTW2/1(ValidPulse) -> Terminator11/1
  DFTW2/4(ValiidFlag) -> [dftvalid2]
  DFTW3/1(ValidPulse) -> Terminator12/1
  DFTW3/4(ValiidFlag) -> [dftvalid3]
  [dftmemWE] -> DFTMem2/7(WE)
  [dftmemWE1] -> DFTMem2/8(WE1)
  [dftmemSel] -> DFTMem2/2(Sel)
  [dftmemStart] -> DFTMem2/1(Start)
  DFTMem2/1(Out1) -> [dftmemDone1]
  DFTW4/2(ImagOutRawLo) -> DFTMem3/3(Src0)
  DFTW4/3(RealOutRawLo) -> DFTMem3/4(Src1)
  DFTW4/5(ImagOutRawHi) -> DFTMem3/5(Src2)
  DFTW4/6(RealOutRawHi) -> DFTMem3/6(Src3)
  DFTW5/2(ImagOutRawLo) -> DFTMem3/9(Src4)
  DFTW5/3(RealOutRawLo) -> DFTMem3/10(Src5)
  DFTW5/5(ImagOutRawHi) -> DFTMem3/11(Src6)
  DFTW5/6(RealOutRawHi) -> DFTMem3/12(Src7)
  DFTW4/1(ValidPulse) -> Terminator13/1
  DFTW4/4(ValiidFlag) -> [dftvalid4]
  DFTW5/1(ValidPulse) -> Terminator14/1
  DFTW5/4(ValiidFlag) -> [dftvalid5]
  [dftmemWE] -> DFTMem3/7(WE)
  [dftmemWE1] -> DFTMem3/8(WE1)
  [dftmemSel] -> DFTMem3/2(Sel)
  [dftmemStart] -> DFTMem3/1(Start)
  DFTMem3/1(Out1) -> [dftmemDone2]
  DFTW6/2(ImagOutRawLo) -> DFTMem4/3(Src0)
  DFTW6/3(RealOutRawLo) -> DFTMem4/4(Src1)
  DFTW6/5(ImagOutRawHi) -> DFTMem4/5(Src2)
  DFTW6/6(RealOutRawHi) -> DFTMem4/6(Src3)
  DFTW7/2(ImagOutRawLo) -> DFTMem4/9(Src4)
  DFTW7/3(RealOutRawLo) -> DFTMem4/10(Src5)
  DFTW7/5(ImagOutRawHi) -> DFTMem4/11(Src6)
  DFTW7/6(RealOutRawHi) -> DFTMem4/12(Src7)
  [dftmemWE] -> DFTMem4/7(WE)
  [dftmemWE1] -> DFTMem4/8(WE1)
  [dftmemSel] -> DFTMem4/2(Sel)
  [dftmemStart] -> DFTMem4/1(Start)
  DFTMem4/1(Out1) -> [dftmemDone3]
  DFTW6/1(ValidPulse) -> Terminator15/1
  DFTW6/4(ValiidFlag) -> [dftvalid6]
  DFTW7/1(ValidPulse) -> Terminator16/1
  DFTW7/4(ValiidFlag) -> [dftvalid7]
  [dftvalid0] -> Logical14/1
  [dftvalid1] -> Logical14/2
  [dftvalid2] -> Logical14/3
  [dftvalid3] -> Logical14/4
  [dftvalid4] -> Logical14/5
  [dftvalid5] -> Logical14/6
  [dftvalid6] -> Logical14/7
  [dftvalid7] -> Logical14/8
  Logical14/1 -> [dftvalidall]
  Logical15/1 -> [dftmemDoneAll]
  [dftmemDone0] -> Logical15/1
  [dftmemDone1] -> Logical15/2
  [dftmemDone2] -> Logical15/3
  [dftmemDone3] -> Logical15/4
  [dftvalidall] -> mainFSM/2
  [dftmemDoneAll] -> mainFSM/1
  mainFSM/4 -> [dftmemWE]
  mainFSM/12 -> [dftmemStart]
  mainFSM/13 -> [dftmemSel]
  adcWaveMem/1(Out1) -> [adcwavememDone]
  [adcwavememStart] -> adcWaveMem/1(Start)
  [adcwavememDone] -> Concat/15
  bit7/1 -> [adcwavememStart]
  bit8/1 -> [adcwavememWE]
  bit9__/1 -> [adcwavememSel]
  controlReg/1(in_reg) -> bit1/1, bit15/1, bit13/1, bit12/1, bit9__/1, bit8/1, bit7/1, bit6/1, bit5/1, bit4/1, bit3/1, bit2/1, bit0/1
  Convert/1 -> Delay1/1
  [adcvalid] -> Concat/14
  adc_mkid_4x/9 -> Logical17/1
  [adcforcesync] -> Logical17/2
  bit12/1 -> [adcforcesync]
  Delay1/1 -> sineNumber/1(out_reg)
  sineNumber/1(sim_out) -> Terminator1/1
  Gateway Out1/1 -> MainFSMScope1/1
  Gateway Out5/1 -> MainFSMScope1/3
  Gateway Out8/1 -> MainFSMScope1/7
  Gateway Out7/1 -> MainFSMScope1/5
  Gateway Out12/1 -> MainFSMScope1/2
  Gateway Out13/1 -> MainFSMScope1/4
  Gateway Out14/1 -> MainFSMScope1/6
  Gateway Out15/1 -> MainFSMScope1/8
  [dftvalidall] -> Gateway Out12/1
  [dftclr] -> Gateway Out5/1
  [dftmemSel] -> Gateway Out13/1
  [dftmemStart] -> Gateway Out7/1
  [dftvalid] -> Gateway Out14/1
  [dftmemWE1] -> Gateway Out8/1
  [trigDftSweep] -> Gateway Out15/1
  adc_mkid_4x/1 -> Mux/3
  adc_mkid_4x/2 -> Mux1/3
  adc_mkid_4x/3 -> Mux7/3
  adc_mkid_4x/4 -> Mux8/3
  adc_mkid_4x/5 -> Mux9/3
  adc_mkid_4x/6 -> Mux10/3
  adc_mkid_4x/7 -> Mux11/3
  adc_mkid_4x/8 -> Mux12/3
  [dacLoopBack] -> Mux/1
  [dacLoopBack] -> Mux1/1
  [dacLoopBack] -> Mux7/1
  [dacLoopBack] -> Mux8/1
  [dacLoopBack] -> Mux9/1
  [dacLoopBack] -> Mux10/1
  [dacLoopBack] -> Mux11/1
  [dacLoopBack] -> Mux12/1
  [cos3] -> fix12_11_/1
  [cos0] -> fix12_11_1/1
  [cos1] -> fix12_11_2/1
  [cos2] -> fix12_11_4/1
  [sin3] -> fix12_11_3/1
  [sin0] -> fix12_11_5/1
  [sin1] -> fix12_11_6/1
  [sin2] -> fix12_11_7/1
  bit13/1 -> [dacLoopBack]
  fix12_11_/1 -> Mux/2
  fix12_11_1/1 -> Mux1/2
  fix12_11_2/1 -> Mux7/2
  fix12_11_4/1 -> Mux8/2
  fix12_11_3/1 -> Mux9/2
  fix12_11_5/1 -> Mux10/2
  fix12_11_6/1 -> Mux11/2
  fix12_11_7/1 -> Mux12/2
  Mux/1 -> [adc_i0]
  [adc_i1] -> DFTW2/1(DataIn)
  [adc_i2] -> DFTW4/1(DataIn)
  [adc_i3] -> DFTW6/1(DataIn)
  [adc_q1] -> DFTW3/1(DataIn)
  [adc_q2] -> DFTW5/1(DataIn)
  Mux11/1 -> [adc_q2]
  [adc_q3] -> DFTW7/1(DataIn)
  Mux12/1 -> [adc_q3]
  [adc_q0] -> DFTW1/1(DataIn)
  [adc_i0] -> DFTW/1(DataIn)
  [adc_i0] -> adcWaveMem/3(Src0)
  adcWaveMem1/1(Out1) -> Terminator17/1
  adcWaveMem3/1(Out1) -> Terminator19/1
  adcWaveMem2/1(Out1) -> Terminator18/1
  Constant/1 -> adcWaveMem/6(WE1)
  [adcwavememSel] -> adcWaveMem/2(Sel)
  [adc_i2] -> adcWaveMem/4(Src1)
  [adcwavememStart] -> adcWaveMem1/1(Start)
  [adc_i1] -> adcWaveMem1/3(Src0)
  Constant17/1 -> adcWaveMem1/6(WE1)
  [adcwavememSel] -> adcWaveMem1/2(Sel)
  [adc_i3] -> adcWaveMem1/4(Src1)
  [adcwavememStart] -> adcWaveMem2/1(Start)
  [adc_q0] -> adcWaveMem2/3(Src0)
  Constant18/1 -> adcWaveMem2/6(WE1)
  [adcwavememSel] -> adcWaveMem2/2(Sel)
  [adc_q2] -> adcWaveMem2/4(Src1)
  [adcwavememStart] -> adcWaveMem3/1(Start)
  [adc_q1] -> adcWaveMem3/3(Src0)
  Constant19/1 -> adcWaveMem3/6(WE1)
  [adcwavememSel] -> adcWaveMem3/2(Sel)
  [adc_q3] -> adcWaveMem3/4(Src1)
  [adcwavememWE] -> adcWaveMem/5(WE)
  [adcwavememWE] -> adcWaveMem1/5(WE)
  [adcwavememWE] -> adcWaveMem2/5(WE)
  [adcwavememWE] -> adcWaveMem3/5(WE)
  SixFourDivLen32p26/1(in_reg) -> [WinFactor]
  [WinFactor] -> DFTW/7(SixFourDivLen)
  [WinFactor] -> DFTW1/7(SixFourDivLen)
  [WinFactor] -> DFTW2/7(SixFourDivLen)
  [WinFactor] -> DFTW3/7(SixFourDivLen)
  Constant20/1 -> SixFourDivLen32p26/1(sim_reg)
  Gateway Out2/1 -> MainFSMScope2/1
  Gateway Out3/1 -> MainFSMScope2/2
  [WinFactor] -> DFTW4/7(SixFourDivLen)
  [WinFactor] -> DFTW5/7(SixFourDivLen)
  [WinFactor] -> DFTW6/7(SixFourDivLen)
  [WinFactor] -> DFTW7/7(SixFourDivLen)
  [cos3] -> Convert/1, dac_mkid_4x/1
  [cos0] -> dac_mkid_4x/2
  [cos1] -> dac_mkid_4x/3
  [cos2] -> dac_mkid_4x/4
  [sin3] -> dac_mkid_4x/5
  [sin0] -> dac_mkid_4x/6
  [sin1] -> dac_mkid_4x/7
  [sin2] -> dac_mkid_4x/8
  gpio_a7/1 -> Terminator20/1
  Counter/1 -> cntbit10/1
  cntbit10/1 -> gpio_a7/1
  [resetDac] -> dac_mkid_4x/13
  bit15/1 -> [resetDac]
